simulink model "top_pipeline_sar_adc_v2"  (R2026a)
settings: Solver=VariableStepAuto
values from neighbouring files (symbols this model uses):
  AMPno = 0.001    [script_MonteCarlo.m]    (also in script_MonteCarlo_v2.m; script_spectrum.m = 0; script_spectrum_v2.m = 0)
  AMPoff = 0.001    [script_MonteCarlo.m]    (also in script_MonteCarlo_v2.m; script_spectrum.m = 0; script_spectrum_v2.m = 0)
  bit_1st = 6    [script_MonteCarlo.m]    (also in script_MonteCarlo_v2.m; script_spectrum.m; script_spectrum_v2.m)
  bit_2nd = 9    [script_MonteCarlo.m]    (also in script_MonteCarlo_v2.m; script_spectrum.m; script_spectrum_v2.m)
  CMPno_1st = 0.0001    [script_MonteCarlo.m]    (also in script_MonteCarlo_v2.m; script_spectrum.m = 0; script_spectrum_v2.m = 0)
  CMPno_2nd = 0.001    [script_MonteCarlo.m]    (also in script_MonteCarlo_v2.m; script_spectrum.m = 0; script_spectrum_v2.m = 0)
  CMPoff_1st = 0.001    [script_MonteCarlo.m]    (also in script_MonteCarlo_v2.m; script_spectrum.m = 0; script_spectrum_v2.m = 0)
  CMPoff_2nd = 0.001    [script_MonteCarlo.m]    (also in script_MonteCarlo_v2.m; script_spectrum.m = 0; script_spectrum_v2.m = 0)
  DAC_1st = DAC_1st_scaled(1 : (bit_1st + 1)) / (2^bit_1st)    [script_MonteCarlo.m]    (also in script_MonteCarlo_v2.m; script_spectrum.m; script_spectrum_v2.m)
  DAC_2nd = 0    [script_MonteCarlo.m]    (also in script_MonteCarlo_v2.m; script_spectrum.m; script_spectrum_v2.m)
settings Model: Creator=오지훈  LastModifiedBy=오지훈

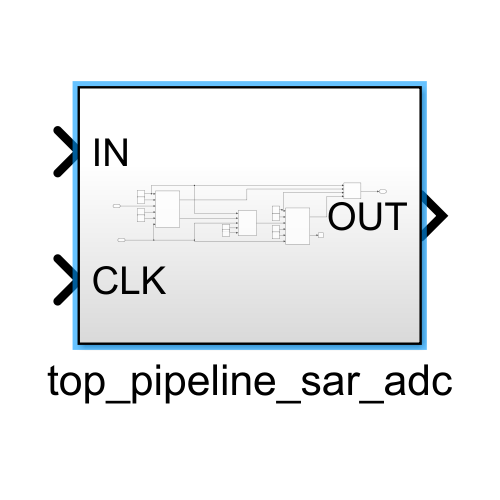
[thumbnail: Simulink's stored preview of the top-level diagram]
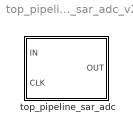
== system top_pipeline_sar_adc_v2 ==
  top_pipeline_sar_adc : Subsystem

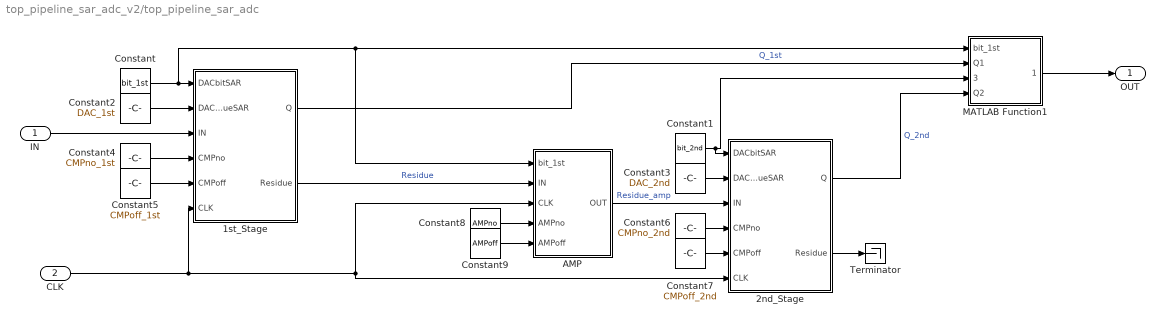
== system top_pipeline_sar_adc_v2/top_pipeline_sar_adc ==
  IN : Inport
  CLK : Inport  Port=2
  1st_Stage : MATLAB Function  TreatAsAtomicUnit=on
  2nd_Stage : MATLAB Function  TreatAsAtomicUnit=on
  AMP : MATLAB Function  TreatAsAtomicUnit=on
  Constant : Constant  Value=bit_1st
  Constant1 : Constant  Value=bit_2nd
  Constant2 : Constant  Value=DAC_1st
  Constant3 : Constant  Value=DAC_2nd
  Constant4 : Constant  Value=CMPno_1st
  Constant5 : Constant  Value=CMPoff_1st
  Constant6 : Constant  Value=CMPno_2nd
  Constant7 : Constant  Value=CMPoff_2nd
  Constant8 : Constant  Value=AMPno
  Constant9 : Constant  Value=AMPoff
  MATLAB Function1 : MATLAB Function  TreatAsAtomicUnit=on
  Terminator : Terminator
  OUT : Outport
  wires:
  Constant2/1 -> 1st_Stage/2(DACvalueSAR)
  2nd_Stage/2(Residue) -> Terminator/1
  1st_Stage/1(Q) -> MATLAB Function1/2(Q1)  "Q_1st"
  Constant4/1 -> 1st_Stage/4(CMPno)
  2nd_Stage/1(Q) -> MATLAB Function1/4(Q2)  "Q_2nd"
  MATLAB Function1/1(Digital_OUT) -> OUT/1
  IN/1 -> 1st_Stage/3(IN)
  Constant/1 -> AMP/1(bit_1st), MATLAB Function1/1(bit_1st), 1st_Stage/1(DACbitSAR)
  1st_Stage/2(Residue) -> AMP/2(IN)  "Residue"
  Constant3/1 -> 2nd_Stage/2(DACvalueSAR)
  Constant6/1 -> 2nd_Stage/4(CMPno)
  Constant1/1 -> 2nd_Stage/1(DACbitSAR), MATLAB Function1/3(bit_2nd)
  Constant5/1 -> 1st_Stage/5(CMPoff)
  Constant7/1 -> 2nd_Stage/5(CMPoff)
  CLK/1 -> 1st_Stage/6(CLK), AMP/3(CLK), 2nd_Stage/6(CLK)
  AMP/1(OUT) -> 2nd_Stage/3(IN)  "Residue_amp"
  Constant8/1 -> AMP/4(AMPno)
  Constant9/1 -> AMP/5(AMPoff)

== matlab function top_pipeline_sar_adc_v2/top_pipeline_sar_adc/1st_Stage ==
  data: DACbitSAR input; Q output; DACvalueSAR input; IN input; CMPno input; CMPoff input; Residue output; CLK input
function [Q, Residue] = SAR_1st(DACbitSAR, DACvalueSAR, IN, CMPno, CMPoff, CLK)
persistent last_CLK Q_hold Residue_hold

if isempty(last_CLK)
    last_CLK = 0;
    Q_hold = 0;
    Residue_hold = 0;
end

if (last_CLK == 0) && (CLK == 1)
    
    current_residue = IN; 
    Q_partial_sum = 0;    % ★ Partial sum을 누적할 변수 초기화
    len_DAC = length(DACvalueSAR); 
    
    for i = 1:DACbitSAR
        CMP_threshold = CMPno * randn(1) + CMPoff;
        
        current_idx = len_DAC - i + 1; 
        current_dac = DACvalueSAR(current_idx);
        
        % 각 비트 자리에 해당하는 이진 가중치 (1, 0.5, 0.25, 0.125 ...)
        bit_weight = 2^(-(i-1)); 
        
        if current_residue >= CMP_threshold
            current_residue = current_residue - current_dac;
            % ★ 비트가 1일 때, 가중치(bit_weight)를 partial sum에 바로 누적
            Q_partial_sum = Q_partial_sum + 1 * bit_weight;
        else
            current_residue = current_residue + current_dac;
            % 비트가 0일 때는 0 * bit_weight 이므로 누적 생략 (혹은 +0)
        end
    end
    
    % ★ 최종 스케일링: [2 곱하기]를 빼고 [1만 빼는] 규칙 적용
    % Virtuoso 수식의 ((VT(MSB) + VT(MSB-1)/2 + ...) - 1) 과 완벽히 매칭됩니다.
    Q_hold = Q_partial_sum - 1;
    
    Residue_hold = current_residue;
end

Q = Q_hold;
Residue = Residue_hold;
last_CLK = CLK;
end

== matlab function top_pipeline_sar_adc_v2/top_pipeline_sar_adc/2nd_Stage ==
  data: DACbitSAR input; Q output; DACvalueSAR input; IN input; CMPno input; CMPoff input; Residue output; CLK input
function [Q, Residue] = SAR_2nd(DACbitSAR, DACvalueSAR, IN, CMPno, CMPoff, CLK)
persistent last_CLK Q_hold Residue_hold

if isempty(last_CLK)
    last_CLK = 0;
    Q_hold = 0;
    Residue_hold = 0;
end

if (last_CLK == 0) && (CLK == 1)
    
    current_residue = IN; 
    Q_partial_sum = 0;    % ★ Partial sum을 누적할 변수 초기화
    len_DAC = length(DACvalueSAR); 
    
    for i = 1:DACbitSAR
        CMP_threshold = CMPno * randn(1) + CMPoff;
        
        current_idx = len_DAC - i + 1; 
        current_dac = DACvalueSAR(current_idx);
        
        % 각 비트 자리에 해당하는 이진 가중치 (1, 0.5, 0.25, 0.125 ...)
        bit_weight = 2^(-(i-1)); 
        
        if current_residue >= CMP_threshold
            current_residue = current_residue - current_dac;
            % ★ 비트가 1일 때, 가중치(bit_weight)를 partial sum에 바로 누적
            Q_partial_sum = Q_partial_sum + 1 * bit_weight;
        else
            current_residue = current_residue + current_dac;
            % 비트가 0일 때는 0 * bit_weight 이므로 누적 생략 (혹은 +0)
        end
    end
    
    % ★ 최종 스케일링: [2 곱하기]를 빼고 [1만 빼는] 규칙 적용
    % Virtuoso 수식의 ((VT(MSB) + VT(MSB-1)/2 + ...) - 1) 과 완벽히 매칭됩니다.
    Q_hold = Q_partial_sum - 1;
    
    Residue_hold = current_residue;
end

Q = Q_hold;
Residue = Residue_hold;
last_CLK = CLK;
end

== matlab function top_pipeline_sar_adc_v2/top_pipeline_sar_adc/AMP ==
  data: bit_1st input; IN input; OUT output; CLK input; AMPno input; AMPoff input
function OUT = AMP(bit_1st, IN, CLK, AMPno, AMPoff)
% AMP Dynamic Amplifier (Single-Ended Version)
%
% Inputs:
%   bit_1st - 1단 해상도 (Gain = 2^bit_1st 계산용)
%   IN      - 단일 입력 신호
%   CLK     - 클록 신호
%   CMPno   - 비교기/증폭기 랜덤 노이즈 표준편차 (Vnstd)
%   CMPoff  - 비교기/증폭기 오프셋 미스매치 전압 (Vos)
%
% Output:
%   OUT     - 증폭된 단일 출력 신호

% 아키텍처 파라미터 설정
Vocm = 0;         % ◀ 입력 신호의 기준점(Common-mode)에 맞게 설정 (예: 0 또는 0.475)
gain = 2^bit_1st;
Vth = 0.5;        % 클록 에지 디텍션 임계값

% 내부 상태 유지를 위한 Persistent 변수
persistent Vin_held Vno ctrl last_CLK initialized
if isempty(initialized)
    Vin_held = 0;
    Vno = 0;
    ctrl = 0;
    last_CLK = CLK;
    initialized = true;
end

% 클록 상승 에지 검출 (Rising Edge)
rising = (last_CLK <= Vth) && (CLK > Vth);

if rising
    % 1. 랜덤 노이즈 전압 생성 (Vnstd * randn)
    Vno = AMPno * randn();
    
    % 2. 상승 에지 순간의 입력 전압 샘플링 및 박제 (Hold)
    Vin_held = IN;
    
    % 3. 증폭 활성화 플래그 ON
    ctrl = 1;
end

% 다음 스텝 에지 검출을 위해 현재 CLK 저장
last_CLK = CLK;

% 4. 기준점(Vocm)으로부터의 변화량에 오프셋(CMPoff)을 더해 증폭한 뒤, 랜덤 노이즈 결합
delta = (Vin_held - Vocm + AMPoff);
OUT = double(Vocm + ctrl * gain * delta + Vno);

end

== matlab function top_pipeline_sar_adc_v2/top_pipeline_sar_adc/MATLAB Function1 ==
  data: bit_1st input; Q1 input; bit_2nd input; Digital_OUT output; Q2 input
function Digital_OUT = fcn(bit_1st, Q1, bit_2nd, Q2)

if (bit_2nd == 0) 
    Digital_OUT = Q1;
else
Digital_OUT = Q1 + Q2*2^(-bit_1st);
end

end
